simulink model "sintesis_metodo_truxal"  (R2020b)
settings: Solver=VariableStepAuto  StartTime=0.0  StopTime=2  RelTol=1e-3
settings Model: Creator=Acer  LastModifiedBy=Acer

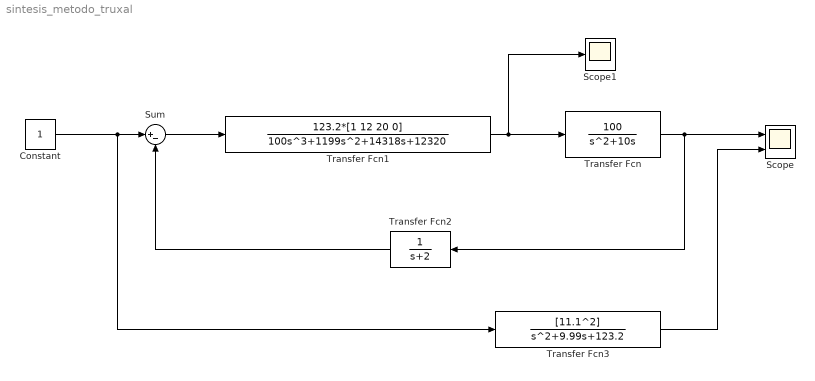
== system sintesis_metodo_truxal ==
  Constant : Constant
  Scope : Scope  NumInputPorts=2
  Scope1 : Scope
  Sum : Sum  Inputs=|+-
  Transfer Fcn : TransferFcn  Numerator=[100]  Denominator=[1 10 0]
  Transfer Fcn1 : TransferFcn  Numerator=123.2*[1 12 20 0]  Denominator=[100 1199 14318 12320]
  Transfer Fcn2 : TransferFcn  Denominator=[1 2]
  Transfer Fcn3 : TransferFcn  Numerator=[11.1^2]  Denominator=[1 9.99 123.2]
  wires:
  Transfer Fcn1/1 -> Scope1/1, Transfer Fcn/1
  Sum/1 -> Transfer Fcn1/1
  Transfer Fcn2/1 -> Sum/2
  Transfer Fcn/1 -> Scope/1, Transfer Fcn2/1
  Transfer Fcn3/1 -> Scope/2
  Constant/1 -> Transfer Fcn3/1, Sum/1
